simulink model "model"  (R2023b)
settings: Solver=VariableStepAuto  StartTime=0.0  StopTime=10.0  RelTol=1e-3
undefined symbols (not defined in the file): a253, a483c26d3aa4, a58537c8, DiscIntNeverNeededParam, magnitude, Newton, Raphson
libraries: simulink x123, slpidlib x33
(part 1 of 5)
settings Model: Creator=OSCAR4  LastModifiedBy=OSCAR4

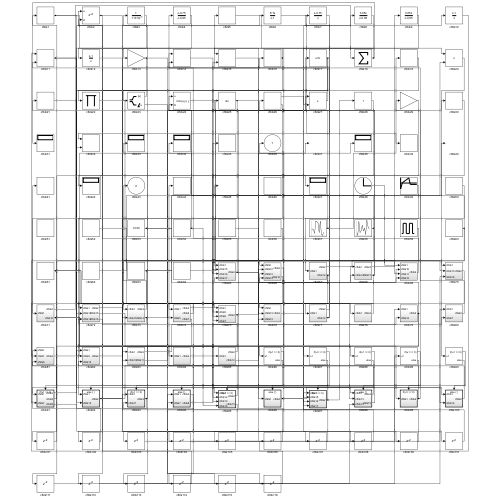
[thumbnail: Simulink's stored preview of the top-level diagram]
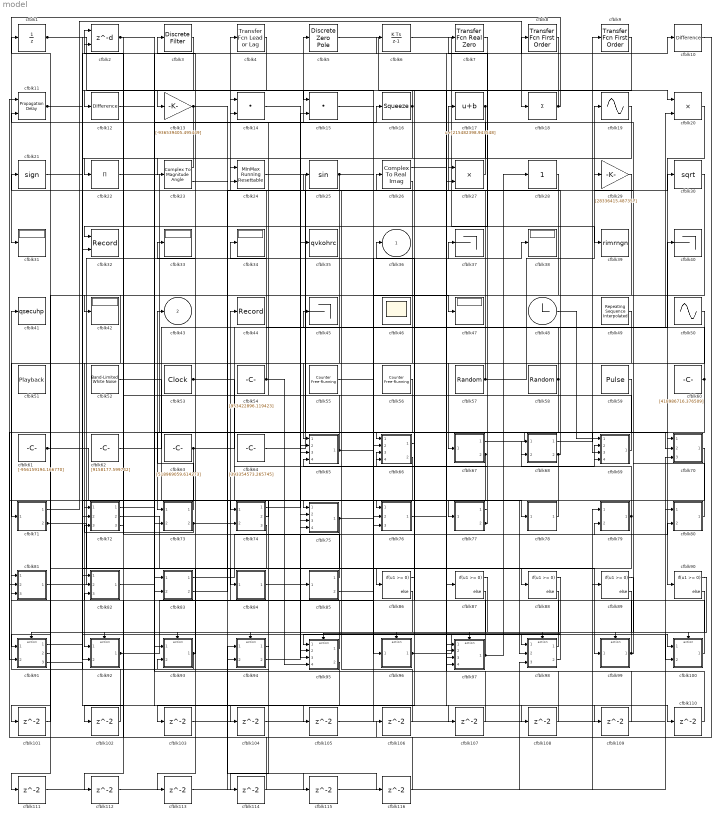
== system model ==
  cfblk1 : UnitDelay  HasFrameUpgradeWarning=on
  cfblk10 : simulink/Discrete/Difference  ICPrevInput=0.0  OutMin=[]  OutMax=[]  OutDataTypeStr=Inherit: Inherit via back propagation  OutDataType=fixdt(1, 16)  OutScaling=2^-10  DoSatur=off
  cfblk100 : Subsystem  TreatAsAtomicUnit=on
  cfblk{101..116} (16 alike) : Delay  SampleTime=1
  cfblk11 : PropagationDelay  SampleTime=1
  cfblk12 : simulink/Discrete/Difference  ICPrevInput=0.0  OutMin=[]  OutMax=[]  OutDataTypeStr=Inherit: Inherit via back propagation  OutDataType=fixdt(1, 16)  OutScaling=2^-10  DoSatur=off
  cfblk13 : Gain  Gain=[-936539405.495449]
  cfblk14 : DotProduct  OutDataTypeStr=Inherit: Inherit via internal rule
  cfblk15 : DotProduct  OutDataTypeStr=Inherit: Inherit via internal rule
  cfblk16 : Squeeze
  cfblk17 : Bias  Bias=[215482398.943548]  SaturateOnIntegerOverflow=off
  cfblk18 : Sum  Inputs=+
  cfblk19 : Sin  TimeSource=Use external signal  SampleTime=0
  cfblk2 : Delay  DelayLengthSource=Input port  SampleTime=1
      settings: InputPortMap=u0,p1
  cfblk20 : Product  Inputs=**
  cfblk21 : Signum
  cfblk22 : Product  Inputs=*
  cfblk23 : ComplexToMagnitudeAngle
  cfblk24 : simulink/Math Operations/MinMax Running Resettable  Function=min  vinit=0.0
  cfblk25 : Trigonometry
  cfblk26 : ComplexToRealImag
  cfblk27 : Product  Inputs=**
  cfblk28 : simulink/Math Operations/Slider Gain  gain=1  low=0  high=2
  cfblk29 : Gain  Gain=[28336415.487357]
  cfblk3 : DiscreteFilter  SampleTime=1
  cfblk30 : Sqrt
  cfblk{31,33..34,38,42,47} (6 alike) : Display
  cfblk32 : Record  FileSettingsInternal="{\"entries\":[{\"content\":{\"excelSettings\":{\"content\":{},\"type\":\"Streamout.ExcelSettings\"}},\"type\":\"Streamout.FileSettingStorage\",\"uuid\":\"\"}],\"packageUris\":[\"http:\\/\\/schema.mathworks.com\\/mf0\\/streamout_blocks\\/R2020a\"],\"version\":\"1.0\"}"  Layout=[1 1]  SignalsInternal="{\"entries\":[{\"content\":{\"signals\":[{\"content\":{\"blockPath\":[],\"dimensions\":[1],\"domain\":\"\",\"lineColor\":\"#a2142f\",\"plots\":[1],\"port\":1,\"signalID\":333,\"signalName\":\"XY Graph:1\"},\"type\":\"RecordBlkView.Signal\",\"uuid\":\"\"},{\"content\":{\"blockPath\":[],\"dimensions\":[1],\"domain\":\"\",\"lineColor\":\"#139fff\",\"plots\":[1],\"port\":2,\"signalID\":336,\"signalName\":\"XY Graph:2\"},\"type\":\"RecordBlkView.Signal\",\"uuid\":\"\"}]},\"type\":\"RecordBlkView.InputSignals\",\"uuid\":\"\"}],\"packageUris\":[\"http:\\/\\/schema.mathworks.com\\/mf0\\/streamout_blocks\\/R2020a\"],\"version\":\"1.0\"}"  VisualizationBindings="{\"xyplotplugin\":{\"info\":[{\"series\":[{\"bindingParametersList\":[{\"parameter\":\"X-Axis\",\"signalID\":333,\"signalName\":\"XY Graph:1\"},{\"parameter\":\"Y-Axis\",\"signalID\":336,\"signalName\":\"XY Graph:2\"}],\"seriesID\":1381}],\"subplotID\":1}]}}"  CompatibilityTag=XY
  cfblk35 : ToWorkspace  VariableName=qvkohrc  SaveFormat=Timeseries  SampleTime=-1
  cfblk37 : Terminator
  cfblk39 : ToWorkspace  VariableName=rimrngn  SaveFormat=Timeseries  SampleTime=-1
  cfblk4 : simulink/Discrete/Transfer Fcn Lead or Lag  PoleZ=0.95  ZeroZ=0.75  ICPrevOutput=0.0  ICPrevInput=0.0  DoSatur=off
  cfblk40 : Terminator
  cfblk41 : ToWorkspace  VariableName=qsecuhp  SaveFormat=Timeseries  SampleTime=-1
  cfblk44 : Record  FileSettingsInternal="{\"entries\":[{\"content\":{\"excelSettings\":{\"content\":{},\"type\":\"Streamout.ExcelSettings\"}},\"type\":\"Streamout.FileSettingStorage\",\"uuid\":\"\"}],\"packageUris\":[\"http:\\/\\/schema.mathworks.com\\/mf0\\/streamout_blocks\\/R2020a\"],\"version\":\"1.0\"}"  SignalsInternal="{\"entries\":[{\"content\":{},\"type\":\"RecordBlkView.InputSignals\",\"uuid\":\"\"}],\"packageUris\":[\"http:\\/\\/schema.mathworks.com\\/mf0\\/streamout_blocks\\/R2020a\"],\"version\":\"1.0\"}"  VisualizationBindings="{\"sparklinesplugin\":{\"info\":[{\"bindingParametersList\":[],\"subplotID\":1}]}}"
  cfblk45 : Terminator
  cfblk46 : Scope
      settings: Floating=on
  cfblk48 : Clock
  cfblk49 : simulink/Sources/Repeating Sequence Interpolated  OutValues=[-862246933.189971, 79795425.555159, 796029637.329822, -177271712.383699, -203597038.742514]  TimeValues=[0 0.1 0.5 0.6 1].'  LookUpMeth=Use Input Above  tsamp=0.01  OutMin=[]  OutMax=[]  OutDataTypeStr=double  OutputDataTypeScalingMode=double  OutDataType=fixdt(0,8)  OutScaling=2^-10
  cfblk5 : DiscreteZeroPole  Poles=[0 0.5]  Gain=1
  cfblk50 : Sin  Amplitude=[622397523.758489]  Bias=[68547005.057914]  SampleTime=0
  cfblk51 : Playback  NumPorts=0  PartName=a58537c8-2575-4d09-a253-a483c26d3aa4
  cfblk52 : simulink/Sources/Band-Limited White Noise  Cov=[7865533069.385715]  Ts=0.1  seed=[9991167842.000000]
  cfblk53 : DigitalClock
  cfblk54 : Constant  Value=[953422896.119423]  SampleTime=1
  cfblk55 : simulink/Sources/Counter Free-Running  NumBits=[8.000000]  tsamp=-1
  cfblk56 : simulink/Sources/Counter Free-Running  NumBits=[25.000000]  tsamp=-1
  cfblk57 : RandomNumber  Mean=[27099.703573]  Variance=[54296.355318]  Seed=[492554018.000000]  SampleTime=0.1
  cfblk58 : UniformRandomNumber  Minimum=[-5476740076.138133]  Maximum=[6087892347.861098]  Seed=[38639628.000000]  SampleTime=0.1
  cfblk59 : DiscretePulseGenerator  PulseType=Time based  Amplitude=[-963513943.362810]  Period=[45867571.560506]  PulseWidth=5  PhaseDelay=[2.000000]
  cfblk6 : DiscreteIntegrator  ICPrevOutput=DiscIntNeverNeededParam  ICPrevScaledInput=DiscIntNeverNeededParam
  cfblk60 : Constant  Value=[418986716.376509]  SampleTime=1
  cfblk61 : Constant  Value=[-956159194.166770]  SampleTime=1
  cfblk62 : Constant  Value=[9158177.599742]  SampleTime=1
  cfblk63 : Constant  Value=[518969059.614273]  SampleTime=1
  cfblk64 : Constant  Value=[393354573.265745]  SampleTime=1
  cfblk65 : Subsystem
  cfblk66 : Subsystem
  cfblk67 : Subsystem
  cfblk68 : Subsystem
  cfblk69 : Subsystem
  cfblk7 : simulink/Discrete/Transfer Fcn Real Zero  ZeroZ=0.75  ICPrevInput=0.0  DoSatur=off
  cfblk70 : Subsystem
  cfblk71 : Subsystem
  cfblk72 : Subsystem
  cfblk73 : Subsystem
  cfblk74 : Subsystem
  cfblk75 : Subsystem
  cfblk76 : Subsystem
  cfblk77 : Subsystem
  cfblk78 : Subsystem
  cfblk79 : Subsystem
  cfblk8 : simulink/Discrete/Transfer Fcn First Order  PoleZ=0.95  ICPrevOutput=0.0  DoSatur=off
  cfblk80 : Subsystem
  cfblk81 : Subsystem
  cfblk82 : Subsystem
  cfblk83 : Subsystem
  cfblk84 : Subsystem
  cfblk85 : Subsystem
  cfblk{86..90} (5 alike) : If  IfExpression=u1 >= 0  SampleTime=1
  cfblk9 : simulink/Discrete/Transfer Fcn First Order  PoleZ=0.95  ICPrevOutput=0.0  DoSatur=off
  cfblk91 : Subsystem  TreatAsAtomicUnit=on
  cfblk92 : Subsystem  TreatAsAtomicUnit=on
  cfblk93 : Subsystem  TreatAsAtomicUnit=on
  cfblk94 : Subsystem  TreatAsAtomicUnit=on
  cfblk95 : Subsystem  TreatAsAtomicUnit=on
  cfblk96 : Subsystem  TreatAsAtomicUnit=on
  cfblk97 : Subsystem  TreatAsAtomicUnit=on
  cfblk98 : Subsystem  TreatAsAtomicUnit=on
  cfblk99 : Subsystem  TreatAsAtomicUnit=on
  cfblk36 : Outport
  cfblk43 : Outport  Port=2
  wires:
  cfblk20/1 -> cfblk90/1
  cfblk81/1(cfblk2) -> cfblk38/1
  cfblk52/1 -> cfblk75/1(cfblk1)
  cfblk27/1 -> cfblk5/1
  cfblk4/1 -> cfblk12/1
  cfblk78/1(cfblk2) -> cfblk76/1(cfblk1)
  cfblk48/1 -> cfblk69/1(cfblk1)
  cfblk7/1 -> cfblk32/1
  cfblk22/1 -> cfblk70/1(cfblk1)
  cfblk57/1 -> cfblk19/1, cfblk14/2
  cfblk99/1(cfblk2) -> cfblk29/1, cfblk81/3(cfblk8)
  cfblk59/1 -> cfblk73/1(cfblk1)
  cfblk14/1 -> cfblk85/1(cfblk1)
  cfblk71/1(cfblk2) -> cfblk18/1
  cfblk82/1(cfblk2) -> cfblk16/1
  cfblk95/1(cfblk2) -> cfblk44/1
  cfblk16/1 -> cfblk13/1, cfblk65/2(cfblk15)
  cfblk55/1 -> cfblk96/1(cfblk1)
  cfblk18/1 -> cfblk31/1, cfblk15/1
  cfblk6/1 -> cfblk39/1
  cfblk70/1(cfblk2) -> cfblk83/2(cfblk10)
  cfblk19/1 -> cfblk42/1
  cfblk58/1 -> cfblk4/1, cfblk91/1(cfblk1)
  cfblk30/1 -> cfblk92/1(cfblk1)
  cfblk24/1 -> cfblk66/1(cfblk1)
  cfblk93/1(cfblk2) -> cfblk41/1, cfblk3/1
  cfblk92/1(cfblk2) -> cfblk66/2(cfblk12), cfblk6/1, cfblk108/1
  cfblk75/1(cfblk2) -> cfblk69/4(cfblk12), cfblk114/1
  cfblk13/1 -> cfblk23/1, cfblk116/1
  cfblk97/1(cfblk2) -> cfblk25/1, cfblk28/1
  cfblk96/1(cfblk2) -> cfblk98/1(cfblk1), cfblk8/1
  cfblk3/1 -> cfblk32/2
  cfblk9/1 -> cfblk86/1
  cfblk91/1(cfblk2) -> cfblk10/1
  cfblk60/1 -> cfblk34/1, cfblk95/3(cfblk13), cfblk65/3(cfblk16)
  cfblk79/1(cfblk2) -> cfblk82/2(cfblk9), cfblk68/1(cfblk1), cfblk101/1
  cfblk1/1 -> cfblk76/2(cfblk13), cfblk75/3(cfblk6)
  cfblk15/1 -> cfblk47/1
  cfblk64/1 -> cfblk17/1
  cfblk68/1(cfblk2) -> cfblk9/1
  cfblk74/1(cfblk2) -> cfblk35/1
  cfblk67/1(cfblk2) -> cfblk70/2(cfblk15)
  cfblk49/1 -> cfblk71/1(cfblk1)
  cfblk12/1 -> cfblk100/1(cfblk1)
  cfblk80/1(cfblk2) -> cfblk11/2
  cfblk98/1(cfblk2) -> cfblk33/1
  cfblk68/2(cfblk15) -> cfblk26/1, cfblk74/2(cfblk5), cfblk21/1
  cfblk85/1(cfblk2) -> cfblk2/1
  cfblk23/1 -> cfblk22/1
  cfblk5/1 -> cfblk20/1
  cfblk100/1(cfblk2) -> cfblk36/1
  cfblk63/1 -> cfblk40/1, cfblk66/4(cfblk14), cfblk91/2(cfblk7)
  cfblk69/1(cfblk2) -> cfblk24/1
  cfblk71/2(cfblk10) -> cfblk88/1, cfblk95/2(cfblk12)
  cfblk98/2(cfblk15) -> cfblk95/1(cfblk1)
  cfblk17/1 -> cfblk92/2(cfblk13), cfblk72/2(cfblk13)
  cfblk85/2(cfblk12) -> cfblk69/2(cfblk10)
  cfblk74/2(cfblk6) -> cfblk72/1(cfblk1)
  cfblk53/1 -> cfblk98/2(cfblk13), cfblk15/2
  cfblk62/1 -> cfblk20/2
  cfblk28/1 -> cfblk75/2(cfblk5)
  cfblk72/2(cfblk15) -> cfblk99/1(cfblk1)
  cfblk25/1 -> cfblk77/1(cfblk1), cfblk65/1(cfblk1)
  cfblk11/1 -> cfblk84/1(cfblk1), cfblk97/4(cfblk17)
  cfblk61/1 -> cfblk78/1(cfblk1), cfblk75/4(cfblk7)
  cfblk91/2(cfblk8) -> cfblk81/1(cfblk1)
  cfblk67/2(cfblk12) -> cfblk66/3(cfblk13), cfblk45/1, cfblk97/3(cfblk16)
  cfblk77/1(cfblk2) -> cfblk7/1
  cfblk83/1(cfblk2) -> cfblk80/2(cfblk7)
  cfblk50/1 -> cfblk67/1(cfblk1)
  cfblk2/1 -> cfblk69/3(cfblk11), cfblk102/1
  cfblk83/2(cfblk11) -> cfblk27/1
  cfblk8/1 -> cfblk27/2
  cfblk73/1(cfblk2) -> cfblk43/1
  cfblk21/1 -> cfblk74/1(cfblk1)
  cfblk65/1(cfblk2) -> cfblk2/2, cfblk37/1, cfblk68/2(cfblk14)
  cfblk76/1(cfblk2) -> cfblk87/1
  cfblk56/1 -> cfblk81/2(cfblk7)
  cfblk26/2 -> cfblk73/2(cfblk11)
  cfblk94/1(cfblk2) -> cfblk93/2(cfblk11)
  cfblk77/2(cfblk12) -> cfblk14/1, cfblk65/4(cfblk17)
  cfblk54/1 -> cfblk24/2, cfblk95/4(cfblk14)
  cfblk73/2(cfblk12) -> cfblk30/1, cfblk72/3(cfblk14)
  cfblk84/1(cfblk2) -> cfblk100/2(cfblk14)
  cfblk94/2(cfblk8) -> cfblk79/2(cfblk14)
  cfblk86/1 -> cfblk91/Action
  cfblk86/2 -> cfblk92/Action
  cfblk87/1 -> cfblk93/Action
  cfblk87/2 -> cfblk94/Action
  cfblk88/1 -> cfblk95/Action
  cfblk88/2 -> cfblk96/Action
  cfblk89/1 -> cfblk97/Action
  cfblk89/2 -> cfblk98/Action
  cfblk90/1 -> cfblk99/Action
  cfblk90/2 -> cfblk100/Action
  cfblk101/1 -> cfblk1/1
  cfblk102/1 -> cfblk82/1(cfblk1)
  cfblk66/1(cfblk2) -> cfblk103/1
  cfblk103/1 -> cfblk80/1(cfblk1)
  cfblk66/2(cfblk15) -> cfblk104/1
  cfblk104/1 -> cfblk89/1
  cfblk95/2(cfblk15) -> cfblk105/1
  cfblk105/1 -> cfblk76/3(cfblk14)
  cfblk10/1 -> cfblk106/1
  cfblk106/1 -> cfblk83/1(cfblk1)
  cfblk91/3(cfblk9) -> cfblk107/1
  cfblk107/1 -> cfblk93/1(cfblk1)
  cfblk108/1 -> cfblk97/2(cfblk15)
  cfblk26/1 -> cfblk109/1
  cfblk109/1 -> cfblk97/1(cfblk1)
  cfblk72/1(cfblk2) -> cfblk110/1
  cfblk110/1 -> cfblk94/1(cfblk1)
  cfblk29/1 -> cfblk111/1
  cfblk111/1 -> cfblk98/3(cfblk14)
  cfblk72/3(cfblk16) -> cfblk112/1
  cfblk112/1 -> cfblk70/3(cfblk16)
  cfblk74/3(cfblk7) -> cfblk113/1
  cfblk113/1 -> cfblk94/2(cfblk7)
  cfblk114/1 -> cfblk11/1
  cfblk23/2 -> cfblk115/1
  cfblk115/1 -> cfblk79/1(cfblk1)
  cfblk116/1 -> cfblk82/3(cfblk10)

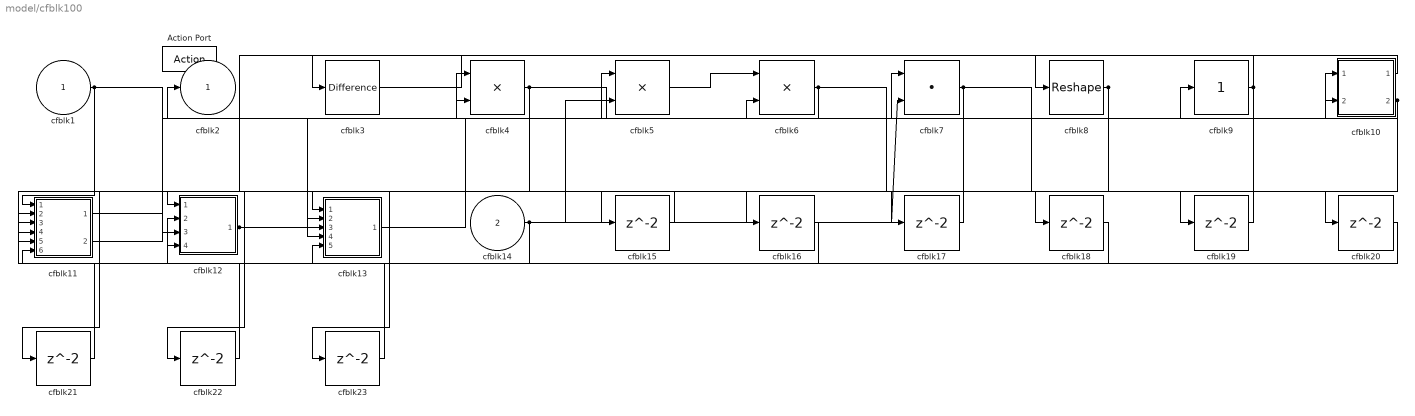
== system model/cfblk100 ==
  cfblk1 : Inport
  cfblk14 : Inport  Port=2
  Action Port : ActionPort  ActionPortLabel=else
  cfblk10 : Subsystem
  cfblk11 : Subsystem
  cfblk12 : Subsystem
  cfblk13 : Subsystem
  cfblk{15..23} (9 alike) : Delay
  cfblk3 : simulink/Discrete/Difference  ICPrevInput=0.0  OutMin=[]  OutMax=[]  OutDataTypeStr=Inherit: Inherit via back propagation  OutDataType=fixdt(1, 16)  OutScaling=2^-10  DoSatur=off
  cfblk4 : Product  Inputs=**
  cfblk5 : Product
  cfblk6 : Product
  cfblk7 : DotProduct  OutDataTypeStr=Inherit: Inherit via internal rule
  cfblk8 : Reshape
  cfblk9 : simulink/Math Operations/Slider Gain  gain=1  low=0  high=2
  cfblk2 : Outport
  wires:
  cfblk13/1(cfblk2) -> cfblk10/1(cfblk1)
  cfblk9/1 -> cfblk12/1(cfblk1), cfblk12/3(cfblk7)
  cfblk14/1 -> cfblk12/2(cfblk6), cfblk5/2, cfblk7/2
  cfblk11/1(cfblk2) -> cfblk9/1
  cfblk7/1 -> cfblk13/1(cfblk1), cfblk20/1
  cfblk10/1(cfblk2) -> cfblk3/1
  cfblk1/1 -> cfblk11/1(cfblk1), cfblk4/1
  cfblk6/1 -> cfblk2/1, cfblk18/1, cfblk19/1
  cfblk11/2(cfblk15) -> cfblk10/2(cfblk16)
  cfblk10/2(cfblk17) -> cfblk5/1, cfblk17/1
  cfblk12/1(cfblk2) -> cfblk7/1, cfblk4/2
  cfblk5/1 -> cfblk6/1
  cfblk8/1 -> cfblk15/1, cfblk16/1
  cfblk3/1 -> cfblk8/1
  cfblk4/1 -> cfblk6/2, cfblk13/4(cfblk16), cfblk21/1, cfblk22/1, cfblk23/1
  cfblk15/1 -> cfblk13/3(cfblk15)
  cfblk16/1 -> cfblk12/4(cfblk8)
  cfblk17/1 -> cfblk13/2(cfblk14)
  cfblk18/1 -> cfblk13/5(cfblk17)
  cfblk19/1 -> cfblk11/3(cfblk11)
  cfblk20/1 -> cfblk11/5(cfblk13)
  cfblk21/1 -> cfblk11/2(cfblk10)
  cfblk22/1 -> cfblk11/4(cfblk12)
  cfblk23/1 -> cfblk11/6(cfblk14)

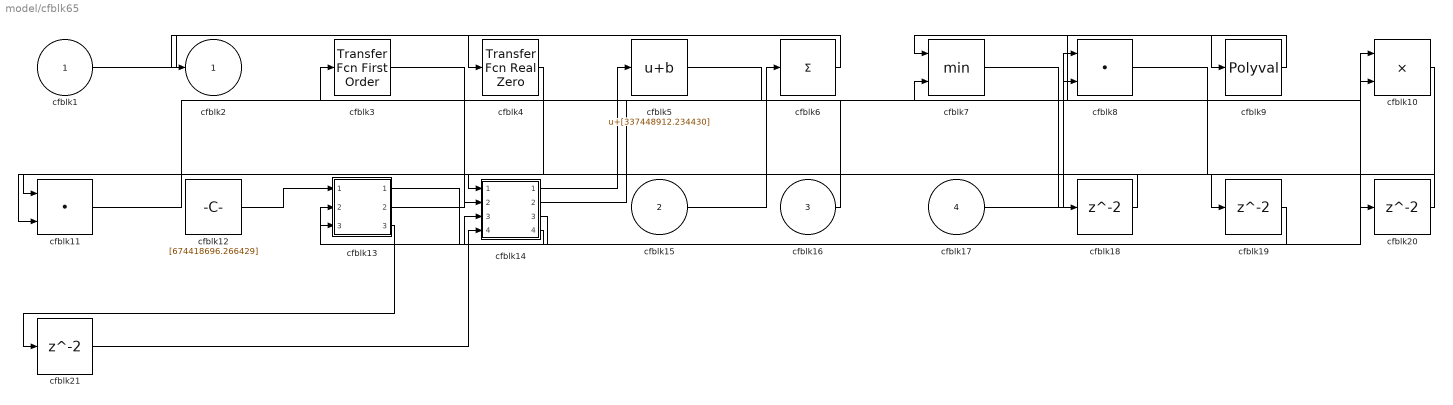
== system model/cfblk65 ==
  cfblk1 : Inport
  cfblk15 : Inport  Port=2
  cfblk16 : Inport  Port=3
  cfblk17 : Inport  Port=4
  cfblk10 : Product
  cfblk11 : DotProduct  OutDataTypeStr=Inherit: Inherit via internal rule
  cfblk12 : Constant  Value=[674418696.266429]  SampleTime=1
  cfblk13 : Subsystem
  cfblk14 : Subsystem
  cfblk{18..21} (4 alike) : Delay  SampleTime=1
  cfblk3 : simulink/Discrete/Transfer Fcn First Order  PoleZ=0.95  ICPrevOutput=0.0  DoSatur=off
  cfblk4 : simulink/Discrete/Transfer Fcn Real Zero  ZeroZ=0.75  ICPrevInput=0.0  DoSatur=off
  cfblk5 : Bias  Bias=[337448912.234430]  SaturateOnIntegerOverflow=off
  cfblk6 : Sum  Inputs=+
  cfblk7 : MinMax  Inputs=2
  cfblk8 : DotProduct  OutDataTypeStr=Inherit: Inherit via internal rule
  cfblk9 : Polyval  Coefs=[ +2.081618890e-019, -1.441693666e-014, +4.719686976e-010, -8.536869453e-006, +1.621573104e-001, -8.087801117e+001 ]
  cfblk2 : Outport
  wires:
  cfblk1/1 -> cfblk4/1
  cfblk11/1 -> cfblk9/1
  cfblk14/1(cfblk2) -> cfblk5/1
  cfblk13/1(cfblk2) -> cfblk10/1
  cfblk6/1 -> cfblk2/1
  cfblk16/1 -> cfblk3/1
  cfblk4/1 -> cfblk11/2
  cfblk15/1 -> cfblk6/1
  cfblk9/1 -> cfblk7/1
  cfblk3/1 -> cfblk14/2(cfblk10)
  cfblk5/1 -> cfblk10/2
  cfblk12/1 -> cfblk13/1(cfblk1)
  cfblk13/2(cfblk14) -> cfblk7/2
  cfblk14/2(cfblk13) -> cfblk8/1
  cfblk17/1 -> cfblk8/2
  cfblk14/3(cfblk14) -> cfblk13/2(cfblk12)
  cfblk14/4(cfblk15) -> cfblk13/3(cfblk13)
  cfblk7/1 -> cfblk18/1
  cfblk18/1 -> cfblk11/1
  cfblk10/1 -> cfblk19/1
  cfblk19/1 -> cfblk14/3(cfblk11)
  cfblk8/1 -> cfblk20/1
  cfblk20/1 -> cfblk14/1(cfblk1)
  cfblk13/3(cfblk15) -> cfblk21/1
  cfblk21/1 -> cfblk14/4(cfblk12)

== system model/cfblk66 ==
  cfblk1 : Inport
  cfblk12 : Inport  Port=2
  cfblk13 : Inport  Port=3
  cfblk14 : Inport  Port=4
  cfblk10 : Subsystem
  cfblk11 : Subsystem
  cfblk16 : Delay  SampleTime=1
  cfblk3 : PropagationDelay  SampleTime=1
  cfblk4 : ComplexToRealImag
  cfblk5 : Product  Inputs=*
  cfblk6 : Trigonometry
  cfblk7 : Constant  Value=[628183486.568107]  SampleTime=1
  cfblk8 : Constant  Value=[532735345.573752]  SampleTime=1
  cfblk9 : Subsystem
  cfblk2 : Outport
  cfblk15 : Outport  Port=2
  wires:
  cfblk12/1 -> cfblk11/1(cfblk1)
  cfblk8/1 -> cfblk2/1
  cfblk10/1(cfblk2) -> cfblk5/1
  cfblk3/1 -> cfblk10/1(cfblk1)
  cfblk6/1 -> cfblk4/1
  cfblk14/1 -> cfblk15/1
  cfblk7/1 -> cfblk3/1
  cfblk9/1(cfblk2) -> cfblk6/1
  cfblk5/1 -> cfblk9/1(cfblk1)
  cfblk11/1(cfblk2) -> cfblk3/2
  cfblk1/1 -> cfblk9/2(cfblk12)
  cfblk11/2(cfblk14) -> cfblk9/3(cfblk13)
  cfblk13/1 -> cfblk9/5(cfblk15)
  cfblk4/1 -> cfblk16/1
  cfblk16/1 -> cfblk9/4(cfblk14)

== system model/cfblk67 ==
  cfblk1 : Inport
  cfblk10 : Subsystem
  cfblk11 : Subsystem
  cfblk13 : Delay  SampleTime=1
  cfblk14 : Delay  SampleTime=1
  cfblk15 : Delay  SampleTime=1
  cfblk3 : simulink/Discrete/Tapped Delay  vinit=0.0  samptime=-1  NumDelays=1  DelayOrder=Oldest  includeCurrent=off
  cfblk4 : simulink/Discrete/Difference  ICPrevInput=0.0  OutMin=[]  OutMax=[]  OutDataTypeStr=Inherit: Inherit via back propagation  OutDataType=fixdt(1, 16)  OutScaling=2^-10  DoSatur=off
  cfblk5 : simulink/Discrete/Transfer Fcn Lead or Lag  PoleZ=0.95  ZeroZ=0.75  ICPrevOutput=0.0  ICPrevInput=0.0  DoSatur=off
  cfblk6 : Signum
  cfblk7 : Sum
  cfblk8 : simulink/Math Operations/MinMax Running Resettable  Function=min  vinit=0.0
  cfblk9 : Constant  Value=[-707875031.415103]  SampleTime=1
  cfblk2 : Outport
  cfblk12 : Outport  Port=2
  wires:
  cfblk7/1 -> cfblk6/1, cfblk14/1
  cfblk3/1 -> cfblk7/1
  cfblk10/1(cfblk2) -> cfblk2/1
  cfblk8/1 -> cfblk3/1, cfblk15/1
  cfblk11/1(cfblk2) -> cfblk8/1
  cfblk9/1 -> cfblk7/2
  cfblk10/2(cfblk13) -> cfblk8/2
  cfblk1/1 -> cfblk5/1, cfblk10/3(cfblk10)
  cfblk10/3(cfblk14) -> cfblk12/1
  cfblk4/1 -> cfblk10/2(cfblk9), cfblk11/2(cfblk7)
  cfblk5/1 -> cfblk4/1, cfblk11/1(cfblk1)
  cfblk6/1 -> cfblk13/1
  cfblk13/1 -> cfblk10/1(cfblk1)
  cfblk14/1 -> cfblk10/5(cfblk12)
  cfblk15/1 -> cfblk10/4(cfblk11)

== system model/cfblk68 ==
  cfblk1 : Inport
  cfblk14 : Inport  Port=2
  cfblk10 : Constant  Value=[-460195986.517128]  SampleTime=1
  cfblk11 : Constant  Value=[291746783.865006]  SampleTime=1
  cfblk12 : Subsystem
  cfblk13 : Subsystem
  cfblk16 : Delay  SampleTime=1
  cfblk17 : Delay  SampleTime=1
  cfblk3 : Delay  ShowEnablePort=on  SampleTime=1
      settings: InputPortMap=u0,e6
  cfblk4 : slpidlib/PID Controller  Controller=PID  Form=Parallel  TimeDomain=Discrete-time  UseExternalTs=off  SampleTime=1  IntegratorMethod=Forward Euler  FilterMethod=Forward Euler  ControllerParametersSource=internal  P=1  I=1  UseKiTs=off  D=0  N=100  UseFilter=on  TunerSelectOption=Transfer Function Based (PID Tuner App)  InitialConditionSource=internal  InitialConditionForIntegrator=0  InitialConditionForFilter=0  DifferentiatorICPrevScaledInput=0  ExternalReset=none  TrackingMode=off  Kt=1  LimitOutput=off  SatLimitsSource=internal  UpperSaturationLimit=inf  LowerSaturationLimit=-inf  LinearizeAsGain=off  AntiWindupMode=none  Kb=1  LimitIntegrator=off  UpperIntegratorSaturationLimit=inf  LowerIntegratorSaturationLimit=-inf  POutMin=[]  POutMax=[]  IOutMin=[]  IOutMax=[]  DOutMin=[]  DOutMax=[]  NOutMin=[]  NOutMax=[]  SumOutMin=[]  SumOutMax=[]  SaturationOutMin=[]  SaturationOutMax=[]  PParamMin=[]  PParamMax=[]  IParamMin=[]  IParamMax=[]  DParamMin=[]  DParamMax=[]  NParamMin=[]  NParamMax=[]  KbParamMin=[]  KbParamMax=[]  KtParamMin=[]  KtParamMax=[]  KbOutMin=[]  KbOutMax=[]  KtOutMin=[]  KtOutMax=[]  IntegratorOutMin=[]  IntegratorOutMax=[]  FilterOutMin=[]  FilterOutMax=[]  SumI1OutMin=[]  SumI1OutMax=[]  SumI2OutMin=[]  SumI2OutMax=[]  SumI3OutMin=[]  SumI3OutMax=[]  SumI4OutMin=[]  SumI4OutMax=[]  SumDOutMin=[]  SumDOutMax=[]  DifferentiatorOutMin=[]  DifferentiatorOutMax=[]  FilterDiffOutCoefMin=[]  FilterDiffOutCoefMax=[]  ReciprocalOutMin=[]  ReciprocalOutMax=[]  SumDenOutMin=[]  SumDenOutMax=[]  SumNumOutMin=[]  SumNumOutMax=[]  DivideOutMin=[]  DivideOutMax=[]  UdiffTsProdOutMin=[]  UdiffTsProdOutMax=[]  NTsProdOutMin=[]  NTsProdOutMax=[]  UintegralTsProdOutMin=[]  UintegralTsProdOutMax=[]  UngainTsProdOutMin=[]  UngainTsProdOutMax=[]  ClampingZeroOutDataTypeStr=Inherit: Inherit via back propagation  ClampingZeroOutMin=[]  ClampingZeroOutMax=[]  FilterDenConstantOutDataTypeStr=Inherit: Inherit via back propagation  FilterDenConstantOutMin=[]  FilterDenConstantOutMax=[]  PCopyOutDataTypeStr=Inherit: Inherit via back propagation  PCopyOutMin=[]  PCopyOutMax=[]  NCopyOutDataTypeStr=Inherit: Inherit via back propagation  NCopyOutMin=[]  NCopyOutMax=[]  IntegratorContinuousStateAttributes=''  IntegratorStateMustResolveToSignalObject=off  IntegratorRTWStateStorageClass=Auto  FilterContinuousStateAttributes=''  FilterStateMustResolveToSignalObject=off  FilterRTWStateStorageClass=Auto  ParallelPVariant=InternalParameters  IdealPVariant=Disabled  IVariant=InternalParameters  DVariant=InternalParameters  IntegratorVariant=Discrete  SatVariant=Disabled  AWVariant=Passthrough  PCopyVariant=Disabled  TRVariant=Disabled  FdbkBlocksVariant=Forward  IdealPFdbkVariant=Disabled  SatFdbkVariant=Disabled  DerivativeFilterVariant=ForwardEulerFilter  NVariant=InternalParameters  NCopyVariant=Disabled  FilterICVariant=InternalICsFilter  IntegratorICVariant=InternalICs  ExternalResetVariant=Disabled  TRSumVariant=Passthrough  SumFdbkVariant=Disabled  SumVariant=Sum_PID  TsampFilterVariant=InternalTs  TsampNgainVariant=Passthrough  TsampIntegralVariant=Disabled_SignalSpec  ExternalSaturationOutDataTypeStr=Inherit: Same as second input
      settings: LibrarySourceBlock=simulink/Discrete/Discrete PID Controller
  cfblk5 : PropagationDelay  SampleTime=1
  cfblk6 : DotProduct  OutDataTypeStr=Inherit: Inherit via internal rule
  cfblk7 : DotProduct  OutDataTypeStr=Inherit: Inherit via internal rule
  cfblk8 : Sqrt  Operator=rSqrt  AlgorithmType=Newton-Raphson
  cfblk9 : Sqrt  Operator=rSqrt  AlgorithmType=Newton-Raphson
  cfblk2 : Outport
  cfblk15 : Outport  Port=2
  wires:
  cfblk3/1 -> cfblk8/1
  cfblk13/1(cfblk2) -> cfblk12/1(cfblk1)
  cfblk8/1 -> cfblk15/1
  cfblk10/1 -> cfblk12/2(cfblk10)
  cfblk13/2(cfblk9) -> cfblk5/1
  cfblk14/1 -> cfblk9/1
  cfblk9/1 -> cfblk2/1, cfblk6/2
  cfblk11/1 -> cfblk4/1, cfblk13/3(cfblk8)
  cfblk1/1 -> cfblk7/1
  cfblk6/1 -> cfblk3/1
  cfblk4/1 -> cfblk7/2
  cfblk7/1 -> cfblk13/1(cfblk1), cfblk13/2(cfblk7), cfblk3/2
  cfblk5/1 -> cfblk16/1, cfblk17/1
  cfblk12/1(cfblk2) -> cfblk5/2
  cfblk12/2(cfblk13) -> cfblk6/1
  cfblk16/1 -> cfblk12/3(cfblk11)
  cfblk17/1 -> cfblk12/4(cfblk12)

== system model/cfblk69 ==
  cfblk1 : Inport
  cfblk10 : Inport  Port=2
  cfblk11 : Inport  Port=3
  cfblk12 : Inport  Port=4
  cfblk{13..16} (4 alike) : Delay  SampleTime=1
  cfblk3 : slpidlib/PID Controller  Controller=PID  Form=Parallel  TimeDomain=Discrete-time  UseExternalTs=off  SampleTime=1  IntegratorMethod=Forward Euler  FilterMethod=Forward Euler  ControllerParametersSource=internal  P=1  I=1  UseKiTs=off  D=0  N=100  UseFilter=on  TunerSelectOption=Transfer Function Based (PID Tuner App)  InitialConditionSource=internal  InitialConditionForIntegrator=0  InitialConditionForFilter=0  DifferentiatorICPrevScaledInput=0  ExternalReset=none  TrackingMode=off  Kt=1  LimitOutput=off  SatLimitsSource=internal  UpperSaturationLimit=inf  LowerSaturationLimit=-inf  LinearizeAsGain=off  AntiWindupMode=none  Kb=1  LimitIntegrator=off  UpperIntegratorSaturationLimit=inf  LowerIntegratorSaturationLimit=-inf  POutMin=[]  POutMax=[]  IOutMin=[]  IOutMax=[]  DOutMin=[]  DOutMax=[]  NOutMin=[]  NOutMax=[]  SumOutMin=[]  SumOutMax=[]  SaturationOutMin=[]  SaturationOutMax=[]  PParamMin=[]  PParamMax=[]  IParamMin=[]  IParamMax=[]  DParamMin=[]  DParamMax=[]  NParamMin=[]  NParamMax=[]  KbParamMin=[]  KbParamMax=[]  KtParamMin=[]  KtParamMax=[]  KbOutMin=[]  KbOutMax=[]  KtOutMin=[]  KtOutMax=[]  IntegratorOutMin=[]  IntegratorOutMax=[]  FilterOutMin=[]  FilterOutMax=[]  SumI1OutMin=[]  SumI1OutMax=[]  SumI2OutMin=[]  SumI2OutMax=[]  SumI3OutMin=[]  SumI3OutMax=[]  SumI4OutMin=[]  SumI4OutMax=[]  SumDOutMin=[]  SumDOutMax=[]  DifferentiatorOutMin=[]  DifferentiatorOutMax=[]  FilterDiffOutCoefMin=[]  FilterDiffOutCoefMax=[]  ReciprocalOutMin=[]  ReciprocalOutMax=[]  SumDenOutMin=[]  SumDenOutMax=[]  SumNumOutMin=[]  SumNumOutMax=[]  DivideOutMin=[]  DivideOutMax=[]  UdiffTsProdOutMin=[]  UdiffTsProdOutMax=[]  NTsProdOutMin=[]  NTsProdOutMax=[]  UintegralTsProdOutMin=[]  UintegralTsProdOutMax=[]  UngainTsProdOutMin=[]  UngainTsProdOutMax=[]  ClampingZeroOutDataTypeStr=Inherit: Inherit via back propagation  ClampingZeroOutMin=[]  ClampingZeroOutMax=[]  FilterDenConstantOutDataTypeStr=Inherit: Inherit via back propagation  FilterDenConstantOutMin=[]  FilterDenConstantOutMax=[]  PCopyOutDataTypeStr=Inherit: Inherit via back propagation  PCopyOutMin=[]  PCopyOutMax=[]  NCopyOutDataTypeStr=Inherit: Inherit via back propagation  NCopyOutMin=[]  NCopyOutMax=[]  IntegratorContinuousStateAttributes=''  IntegratorStateMustResolveToSignalObject=off  IntegratorRTWStateStorageClass=Auto  FilterContinuousStateAttributes=''  FilterStateMustResolveToSignalObject=off  FilterRTWStateStorageClass=Auto  ParallelPVariant=InternalParameters  IdealPVariant=Disabled  IVariant=InternalParameters  DVariant=InternalParameters  IntegratorVariant=Discrete  SatVariant=Disabled  AWVariant=Passthrough  PCopyVariant=Disabled  TRVariant=Disabled  FdbkBlocksVariant=Forward  IdealPFdbkVariant=Disabled  SatFdbkVariant=Disabled  DerivativeFilterVariant=ForwardEulerFilter  NVariant=InternalParameters  NCopyVariant=Disabled  FilterICVariant=InternalICsFilter  IntegratorICVariant=InternalICs  ExternalResetVariant=Disabled  TRSumVariant=Passthrough  SumFdbkVariant=Disabled  SumVariant=Sum_PID  TsampFilterVariant=InternalTs  TsampNgainVariant=Passthrough  TsampIntegralVariant=Disabled_SignalSpec  ExternalSaturationOutDataTypeStr=Inherit: Same as second input
      settings: LibrarySourceBlock=simulink/Discrete/Discrete PID Controller
  cfblk4 : Math  Operator=log
  cfblk5 : Trigonometry
  cfblk6 : UnaryMinus
  cfblk7 : Subsystem
  cfblk8 : Subsystem
  cfblk9 : Subsystem
  cfblk2 : Outport
  wires:
  cfblk3/1 -> cfblk6/1
  cfblk7/1(cfblk2) -> cfblk2/1
  cfblk11/1 -> cfblk7/1(cfblk1)
  cfblk12/1 -> cfblk7/2(cfblk9)
  cfblk8/1(cfblk2) -> cfblk3/1
  cfblk10/1 -> cfblk8/1(cfblk1)
  cfblk5/1 -> cfblk4/1
  cfblk8/2(cfblk12) -> cfblk9/1(cfblk1)
  cfblk9/1(cfblk2) -> cfblk5/1
  cfblk1/1 -> cfblk8/5(cfblk11)
  cfblk4/1 -> cfblk7/3(cfblk10)
  cfblk6/1 -> cfblk13/1
  cfblk13/1 -> cfblk8/2(cfblk8)
  cfblk7/2(cfblk11) -> cfblk14/1
  cfblk14/1 -> cfblk9/2(cfblk12)
  cfblk9/2(cfblk13) -> cfblk15/1
  cfblk15/1 -> cfblk8/3(cfblk9)
  cfblk9/3(cfblk14) -> cfblk16/1
  cfblk16/1 -> cfblk8/4(cfblk10)

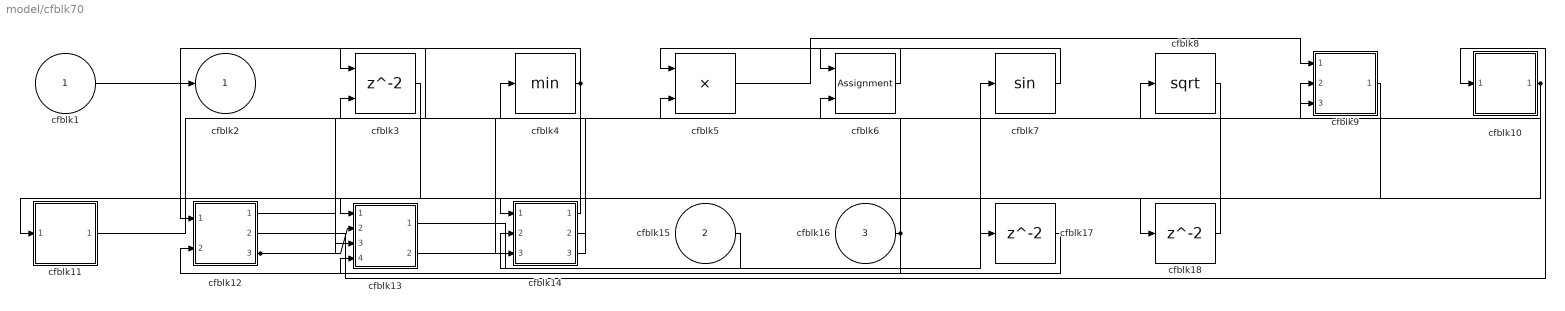
== system model/cfblk70 ==
  cfblk1 : Inport
  cfblk15 : Inport  Port=2
  cfblk16 : Inport  Port=3
  cfblk10 : Subsystem
  cfblk11 : Subsystem
  cfblk12 : Subsystem
  cfblk13 : Subsystem
  cfblk14 : Subsystem
  cfblk17 : Delay  SampleTime=1
  cfblk18 : Delay  SampleTime=1
  cfblk3 : Delay  ShowEnablePort=on  SampleTime=1
      settings: InputPortMap=u0,e6
  cfblk4 : MinMax
  cfblk5 : Product
  cfblk6 : Assignment  DiagnosticForDimensions=Warning  IndexOptions=Index vector (dialog)  Indices=1  OutputSizes=1
  cfblk7 : Trigonometry
  cfblk8 : Sqrt
  cfblk9 : Subsystem
  cfblk2 : Outport
  wires:
  cfblk3/1 -> cfblk11/1(cfblk1)
  cfblk14/1(cfblk2) -> cfblk3/1
  cfblk7/1 -> cfblk6/1
  cfblk13/1(cfblk2) -> cfblk7/1
  cfblk11/1(cfblk2) -> cfblk6/2
  cfblk16/1 -> cfblk3/2, cfblk13/4(cfblk12)
  cfblk1/1 -> cfblk12/1(cfblk1)
  cfblk4/1 -> cfblk2/1, cfblk13/3(cfblk11)
  cfblk13/2(cfblk13) -> cfblk8/1
  cfblk15/1 -> cfblk14/2(cfblk12)
  cfblk10/1(cfblk2) -> cfblk14/3(cfblk13), cfblk5/2
  cfblk5/1 -> cfblk9/1(cfblk1)
  cfblk14/2(cfblk14) -> cfblk4/1
  cfblk6/1 -> cfblk5/1
  cfblk14/3(cfblk15) -> cfblk13/1(cfblk1)
  cfblk12/1(cfblk2) -> cfblk9/2(cfblk10)
  cfblk12/2(cfblk10) -> cfblk10/1(cfblk1)
  cfblk12/3(cfblk11) -> cfblk13/2(cfblk10), cfblk9/3(cfblk11)
  cfblk9/1(cfblk2) -> cfblk17/1
  cfblk17/1 -> cfblk12/2(cfblk9)
  cfblk8/1 -> cfblk18/1
  cfblk18/1 -> cfblk14/1(cfblk1)

== system model/cfblk71 ==
  cfblk1 : Inport
  cfblk{11..14} (4 alike) : Delay  SampleTime=1
  cfblk3 : DiscreteIntegrator  ICPrevOutput=DiscIntNeverNeededParam  ICPrevScaledInput=DiscIntNeverNeededParam
  cfblk4 : ComplexToRealImag
  cfblk5 : Sin  TimeSource=Use external signal  SampleTime=0
  cfblk6 : DotProduct  OutDataTypeStr=Inherit: Inherit via internal rule
  cfblk7 : UnaryMinus
  cfblk8 : Subsystem
  cfblk9 : Subsystem
  cfblk2 : Outport
  cfblk10 : Outport  Port=2
  wires:
  cfblk5/1 -> cfblk12/1, cfblk13/1
  cfblk3/1 -> cfblk4/1
  cfblk8/1(cfblk2) -> cfblk10/1
  cfblk6/1 -> cfblk5/1, cfblk3/1
  cfblk7/1 -> cfblk9/1(cfblk1)
  cfblk1/1 -> cfblk7/1
  cfblk8/3(cfblk14) -> cfblk6/2
  cfblk4/2 -> cfblk2/1
  cfblk9/1(cfblk2) -> cfblk8/1(cfblk1)
  cfblk9/2(cfblk15) -> cfblk8/2(cfblk11)
  cfblk8/2(cfblk13) -> cfblk11/1
  cfblk11/1 -> cfblk9/2(cfblk13)
  cfblk12/1 -> cfblk6/1
  cfblk13/1 -> cfblk8/3(cfblk12)
  cfblk4/1 -> cfblk14/1
  cfblk14/1 -> cfblk9/3(cfblk14)

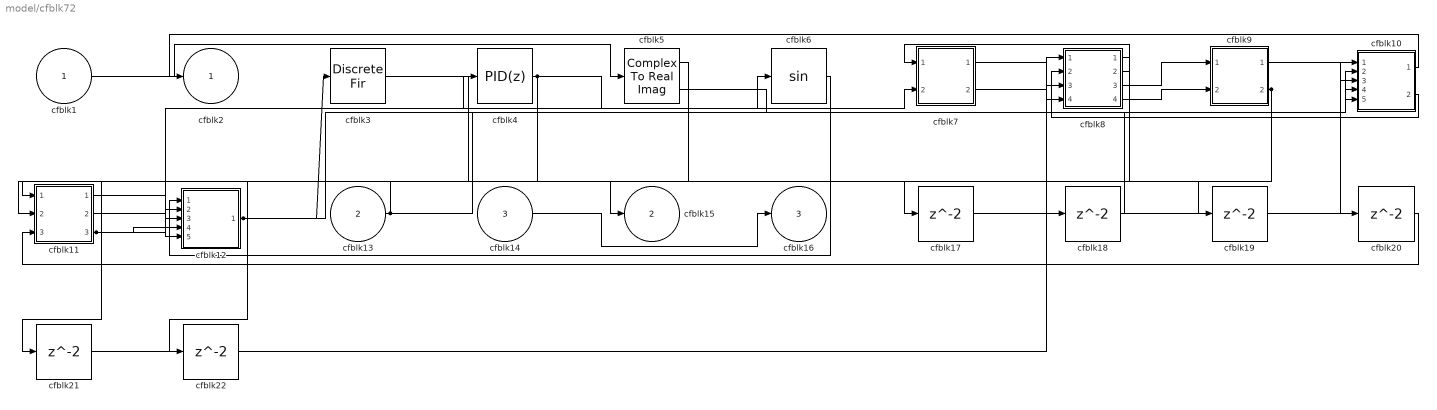
== system model/cfblk72 ==
  cfblk1 : Inport
  cfblk13 : Inport  Port=2
  cfblk14 : Inport  Port=3
  cfblk10 : Subsystem
  cfblk11 : Subsystem
  cfblk12 : Subsystem
  cfblk{17..22} (6 alike) : Delay  SampleTime=1
  cfblk3 : DiscreteFir  SampleTime=1
  cfblk4 : slpidlib/PID Controller  Controller=PID  Form=Parallel  TimeDomain=Discrete-time  UseExternalTs=off  SampleTime=1  IntegratorMethod=Forward Euler  FilterMethod=Forward Euler  ControllerParametersSource=internal  P=1  I=1  UseKiTs=off  D=0  N=100  UseFilter=on  TunerSelectOption=Transfer Function Based (PID Tuner App)  InitialConditionSource=internal  InitialConditionForIntegrator=0  InitialConditionForFilter=0  DifferentiatorICPrevScaledInput=0  ExternalReset=none  TrackingMode=off  Kt=1  LimitOutput=off  SatLimitsSource=internal  UpperSaturationLimit=inf  LowerSaturationLimit=-inf  LinearizeAsGain=off  AntiWindupMode=none  Kb=1  LimitIntegrator=off  UpperIntegratorSaturationLimit=inf  LowerIntegratorSaturationLimit=-inf  POutMin=[]  POutMax=[]  IOutMin=[]  IOutMax=[]  DOutMin=[]  DOutMax=[]  NOutMin=[]  NOutMax=[]  SumOutMin=[]  SumOutMax=[]  SaturationOutMin=[]  SaturationOutMax=[]  PParamMin=[]  PParamMax=[]  IParamMin=[]  IParamMax=[]  DParamMin=[]  DParamMax=[]  NParamMin=[]  NParamMax=[]  KbParamMin=[]  KbParamMax=[]  KtParamMin=[]  KtParamMax=[]  KbOutMin=[]  KbOutMax=[]  KtOutMin=[]  KtOutMax=[]  IntegratorOutMin=[]  IntegratorOutMax=[]  FilterOutMin=[]  FilterOutMax=[]  SumI1OutMin=[]  SumI1OutMax=[]  SumI2OutMin=[]  SumI2OutMax=[]  SumI3OutMin=[]  SumI3OutMax=[]  SumI4OutMin=[]  SumI4OutMax=[]  SumDOutMin=[]  SumDOutMax=[]  DifferentiatorOutMin=[]  DifferentiatorOutMax=[]  FilterDiffOutCoefMin=[]  FilterDiffOutCoefMax=[]  ReciprocalOutMin=[]  ReciprocalOutMax=[]  SumDenOutMin=[]  SumDenOutMax=[]  SumNumOutMin=[]  SumNumOutMax=[]  DivideOutMin=[]  DivideOutMax=[]  UdiffTsProdOutMin=[]  UdiffTsProdOutMax=[]  NTsProdOutMin=[]  NTsProdOutMax=[]  UintegralTsProdOutMin=[]  UintegralTsProdOutMax=[]  UngainTsProdOutMin=[]  UngainTsProdOutMax=[]  ClampingZeroOutDataTypeStr=Inherit: Inherit via back propagation  ClampingZeroOutMin=[]  ClampingZeroOutMax=[]  FilterDenConstantOutDataTypeStr=Inherit: Inherit via back propagation  FilterDenConstantOutMin=[]  FilterDenConstantOutMax=[]  PCopyOutDataTypeStr=Inherit: Inherit via back propagation  PCopyOutMin=[]  PCopyOutMax=[]  NCopyOutDataTypeStr=Inherit: Inherit via back propagation  NCopyOutMin=[]  NCopyOutMax=[]  IntegratorContinuousStateAttributes=''  IntegratorStateMustResolveToSignalObject=off  IntegratorRTWStateStorageClass=Auto  FilterContinuousStateAttributes=''  FilterStateMustResolveToSignalObject=off  FilterRTWStateStorageClass=Auto  ParallelPVariant=InternalParameters  IdealPVariant=Disabled  IVariant=InternalParameters  DVariant=InternalParameters  IntegratorVariant=Discrete  SatVariant=Disabled  AWVariant=Passthrough  PCopyVariant=Disabled  TRVariant=Disabled  FdbkBlocksVariant=Forward  IdealPFdbkVariant=Disabled  SatFdbkVariant=Disabled  DerivativeFilterVariant=ForwardEulerFilter  NVariant=InternalParameters  NCopyVariant=Disabled  FilterICVariant=InternalICsFilter  IntegratorICVariant=InternalICs  ExternalResetVariant=Disabled  TRSumVariant=Passthrough  SumFdbkVariant=Disabled  SumVariant=Sum_PID  TsampFilterVariant=InternalTs  TsampNgainVariant=Passthrough  TsampIntegralVariant=Disabled_SignalSpec  ExternalSaturationOutDataTypeStr=Inherit: Same as second input
      settings: LibrarySourceBlock=simulink/Discrete/Discrete PID Controller
  cfblk5 : ComplexToRealImag
  cfblk6 : Trigonometry
  cfblk7 : Subsystem
  cfblk8 : Subsystem
  cfblk9 : Subsystem
  cfblk2 : Outport
  cfblk15 : Outport  Port=2
  cfblk16 : Outport  Port=3
  wires:
  cfblk1/1 -> cfblk5/1
  cfblk3/1 -> cfblk15/1
  cfblk4/1 -> cfblk6/1, cfblk12/3(cfblk11), cfblk12/5(cfblk13)
  cfblk6/1 -> cfblk12/1(cfblk1)
  cfblk14/1 -> cfblk16/1
  cfblk11/1(cfblk2) -> cfblk12/2(cfblk10)
  cfblk10/1(cfblk2) -> cfblk2/1
  cfblk5/1 -> cfblk11/1(cfblk1)
  cfblk12/1(cfblk2) -> cfblk3/1, cfblk10/4(cfblk11)
  cfblk5/2 -> cfblk10/2(cfblk9)
  cfblk8/2(cfblk13) -> cfblk7/1(cfblk1)
  cfblk13/1 -> cfblk11/2(cfblk13), cfblk10/5(cfblk12)
  cfblk10/2(cfblk13) -> cfblk8/2(cfblk10)
  cfblk11/2(cfblk15) -> cfblk7/2(cfblk9)
  cfblk9/2(cfblk12) -> cfblk21/1, cfblk22/1
  cfblk11/3(cfblk16) -> cfblk4/1, cfblk12/4(cfblk12)
  cfblk8/3(cfblk14) -> cfblk9/1(cfblk1)
  cfblk8/4(cfblk15) -> cfblk9/2(cfblk11)
  cfblk8/1(cfblk2) -> cfblk17/1
  cfblk17/1 -> cfblk10/1(cfblk1)
  cfblk7/1(cfblk2) -> cfblk18/1
  cfblk18/1 -> cfblk8/1(cfblk1)
  cfblk7/2(cfblk10) -> cfblk19/1
  cfblk19/1 -> cfblk10/3(cfblk10)
  cfblk9/1(cfblk2) -> cfblk20/1
  cfblk20/1 -> cfblk11/3(cfblk14)
  cfblk21/1 -> cfblk8/3(cfblk11)
  cfblk22/1 -> cfblk8/4(cfblk12)

== system model/cfblk73 ==
  cfblk1 : Inport
  cfblk11 : Inport  Port=2
  cfblk10 : Subsystem
  cfblk{13..16} (4 alike) : Delay  SampleTime=1
  cfblk3 : simulink/Discrete/Transfer Fcn Lead or Lag  PoleZ=0.95  ZeroZ=0.75  ICPrevOutput=0.0  ICPrevInput=0.0  DoSatur=off
  cfblk4 : DiscreteZeroPole  Poles=[0 0.5]  Gain=1
  cfblk5 : Sqrt
  cfblk6 : Constant  Value=[251991001.423929]  SampleTime=1
  cfblk7 : Subsystem
  cfblk8 : Subsystem
  cfblk9 : Subsystem
  cfblk2 : Outport
  cfblk12 : Outport  Port=2
  wires:
  cfblk11/1 -> cfblk10/1(cfblk1), cfblk8/4(cfblk11)
  cfblk5/1 -> cfblk13/1, cfblk14/1
  cfblk8/1(cfblk2) -> cfblk3/1
  cfblk1/1 -> cfblk7/2(cfblk13)
  cfblk4/1 -> cfblk5/1
  cfblk6/1 -> cfblk10/2(cfblk8)
  cfblk7/1(cfblk2) -> cfblk12/1
  cfblk10/1(cfblk2) -> cfblk4/1
  cfblk3/1 -> cfblk2/1, cfblk15/1
  cfblk10/2(cfblk11) -> cfblk8/1(cfblk1)
  cfblk7/2(cfblk15) -> cfblk9/1(cfblk1)
  cfblk9/1(cfblk2) -> cfblk10/3(cfblk9)
  cfblk7/3(cfblk16) -> cfblk10/4(cfblk10)
  cfblk9/2(cfblk11) -> cfblk8/2(cfblk9)
  cfblk9/3(cfblk12) -> cfblk8/3(cfblk10)
  cfblk13/1 -> cfblk7/1(cfblk1)
  cfblk14/1 -> cfblk9/2(cfblk9)
  cfblk15/1 -> cfblk9/3(cfblk10)
  cfblk8/2(cfblk12) -> cfblk16/1
  cfblk16/1 -> cfblk7/3(cfblk14)

== system model/cfblk74 ==
  cfblk1 : Inport
  cfblk5 : Inport  Port=2
  cfblk3 : DiscreteZeroPole  Poles=[0 0.5]  Gain=1
  cfblk4 : Subsystem
  cfblk2 : Outport
  cfblk6 : Outport  Port=2
  cfblk7 : Outport  Port=3
  wires:
  cfblk5/1 -> cfblk4/1(cfblk1), cfblk3/1
  cfblk1/1 -> cfblk6/1
  cfblk4/1(cfblk2) -> cfblk7/1
  cfblk3/1 -> cfblk2/1

== system model/cfblk75 ==
  cfblk1 : Inport
  cfblk5 : Inport  Port=2
  cfblk6 : Inport  Port=3
  cfblk7 : Inport  Port=4
  cfblk{10..13} (4 alike) : Delay  SampleTime=1
  cfblk3 : Subsystem
  cfblk4 : If  IfExpression=u1 >= 0  SampleTime=1
  cfblk8 : Subsystem  TreatAsAtomicUnit=on
  cfblk9 : Subsystem  TreatAsAtomicUnit=on
  cfblk2 : Outport
  wires:
  cfblk5/1 -> cfblk9/1(cfblk1)
  cfblk7/1 -> cfblk4/1
  cfblk1/1 -> cfblk3/1(cfblk1)
  cfblk6/1 -> cfblk8/1(cfblk1)
  cfblk3/1(cfblk2) -> cfblk9/2(cfblk13)
  cfblk9/1(cfblk2) -> cfblk8/2(cfblk10)
  cfblk9/3(cfblk15) -> cfblk8/3(cfblk11)
  cfblk9/4(cfblk16) -> cfblk12/1, cfblk13/1
  cfblk8/1(cfblk2) -> cfblk2/1
  cfblk3/2(cfblk17) -> cfblk8/4(cfblk12)
  cfblk4/1 -> cfblk8/Action
  cfblk4/2 -> cfblk9/Action
  cfblk8/2(cfblk13) -> cfblk10/1
  cfblk10/1 -> cfblk3/4(cfblk15)
  cfblk9/2(cfblk14) -> cfblk11/1
  cfblk11/1 -> cfblk3/2(cfblk13)
  cfblk12/1 -> cfblk3/3(cfblk14)
  cfblk13/1 -> cfblk3/5(cfblk16)

== system model/cfblk76 ==
  cfblk1 : Inport
  cfblk13 : Inport  Port=2
  cfblk14 : Inport  Port=3
  cfblk10 : Subsystem
  cfblk11 : Subsystem
  cfblk12 : Subsystem
  cfblk15 : Delay  SampleTime=1
  cfblk16 : Delay  SampleTime=1
  cfblk3 : simulink/Discrete/Tapped Delay  vinit=0.0  samptime=-1  NumDelays=1  DelayOrder=Oldest  includeCurrent=off
  cfblk4 : simulink/Discrete/Difference  ICPrevInput=0.0  OutMin=[]  OutMax=[]  OutDataTypeStr=Inherit: Inherit via back propagation  OutDataType=fixdt(1, 16)  OutScaling=2^-10  DoSatur=off
  cfblk5 : DiscreteZeroPole  Poles=[0 0.5]  Gain=1
  cfblk6 : simulink/Math Operations/Slider Gain  gain=1  low=0  high=2
  cfblk7 : UnaryMinus
  cfblk8 : PermuteDimensions
  cfblk9 : Subsystem
  cfblk2 : Outport
  wires:
  cfblk7/1 -> cfblk12/1(cfblk1)
  cfblk8/1 -> cfblk10/1(cfblk1)
  cfblk4/1 -> cfblk2/1
  cfblk1/1 -> cfblk9/1(cfblk1)
  cfblk3/1 -> cfblk12/3(cfblk8)
  cfblk13/1 -> cfblk10/2(cfblk7)
  cfblk11/1(cfblk2) -> cfblk5/1
  cfblk14/1 -> cfblk7/1
  cfblk12/1(cfblk2) -> cfblk8/1
  cfblk10/2(cfblk8) -> cfblk11/1(cfblk1)
  cfblk6/1 -> cfblk4/1
  cfblk11/3(cfblk7) -> cfblk6/1
  cfblk10/1(cfblk2) -> cfblk15/1
  cfblk15/1 -> cfblk12/2(cfblk7)
  cfblk11/2(cfblk6) -> cfblk16/1
  cfblk16/1 -> cfblk3/1

== system model/cfblk77 ==
  cfblk1 : Inport
  cfblk10 : Subsystem
  cfblk11 : Subsystem
  cfblk{13..17} (5 alike) : Delay  SampleTime=1
  cfblk3 : Delay  ShowEnablePort=on  SampleTime=1
      settings: InputPortMap=u0,e6
  cfblk4 : UnaryMinus
  cfblk5 : MinMax  Function=max
  cfblk6 : Sqrt
  cfblk7 : simulink/Math Operations/MinMax Running Resettable  Function=min  vinit=0.0
  cfblk8 : Subsystem
  cfblk9 : Subsystem
  cfblk2 : Outport
  cfblk12 : Outport  Port=2
  wires:
  cfblk10/1(cfblk2) -> cfblk2/1
  cfblk9/1(cfblk2) -> cfblk3/1
  cfblk11/1(cfblk2) -> cfblk6/1
  cfblk6/1 -> cfblk8/1(cfblk1), cfblk16/1
  cfblk1/1 -> cfblk9/2(cfblk11)
  cfblk4/1 -> cfblk5/1
  cfblk10/2(cfblk11) -> cfblk11/1(cfblk1)
  cfblk9/2(cfblk13) -> cfblk3/2
  cfblk11/2(cfblk7) -> cfblk8/2(cfblk12), cfblk7/1
  cfblk10/3(cfblk12) -> cfblk4/1, cfblk12/1
  cfblk3/1 -> cfblk10/4(cfblk10), cfblk13/1
  cfblk8/1(cfblk2) -> cfblk7/2, cfblk14/1
  cfblk13/1 -> cfblk9/3(cfblk12)
  cfblk14/1 -> cfblk10/2(cfblk8)
  cfblk7/1 -> cfblk15/1
  cfblk15/1 -> cfblk10/1(cfblk1)
  cfblk16/1 -> cfblk10/3(cfblk9)
  cfblk5/1 -> cfblk17/1
  cfblk17/1 -> cfblk9/1(cfblk1)

== system model/cfblk78 ==
  cfblk1 : Inport
  cfblk3 : Delay  SampleTime=1
  cfblk4 : Reshape
  cfblk5 : Sum  Inputs=+
  cfblk6 : Subsystem
  cfblk7 : Subsystem
  cfblk8 : Delay  SampleTime=1
  cfblk2 : Outport
  wires:
  cfblk1/1 -> cfblk4/1
  cfblk7/1(cfblk2) -> cfblk6/1(cfblk1)
  cfblk4/1 -> cfblk5/1, cfblk6/3(cfblk9)
  cfblk6/1(cfblk2) -> cfblk2/1
  cfblk5/1 -> cfblk7/2(cfblk8)
  cfblk7/2(cfblk9) -> cfblk3/1
  cfblk3/1 -> cfblk6/2(cfblk8)
  cfblk6/2(cfblk10) -> cfblk8/1
  cfblk8/1 -> cfblk7/1(cfblk1)

== system model/cfblk79 ==
  cfblk1 : Inport
  cfblk14 : Inport  Port=2
  cfblk10 : Subsystem
  cfblk11 : Subsystem
  cfblk12 : Subsystem
  cfblk13 : Subsystem
  cfblk15 : Delay  SampleTime=1
  cfblk16 : Delay  SampleTime=1
  cfblk3 : simulink/Discrete/Difference  ICPrevInput=0.0  OutMin=[]  OutMax=[]  OutDataTypeStr=Inherit: Inherit via back propagation  OutDataType=fixdt(1, 16)  OutScaling=2^-10  DoSatur=off
  cfblk4 : Delay  DelayLengthSource=Input port  SampleTime=1
      settings: InputPortMap=u0,p1
  cfblk5 : Delay  ShowEnablePort=on  SampleTime=1
      settings: InputPortMap=u0,e6
  cfblk6 : Delay  ShowEnablePort=on  SampleTime=1
      settings: InputPortMap=u0,e6
  cfblk7 : Gain  Gain=[-633947602.308004]
  cfblk8 : Constant  Value=[6845603.135488]  SampleTime=1
  cfblk9 : Subsystem
  cfblk2 : Outport
  wires:
  cfblk13/1(cfblk2) -> cfblk6/1
  cfblk8/1 -> cfblk12/1(cfblk1)
  cfblk5/1 -> cfblk7/1
  cfblk4/1 -> cfblk11/1(cfblk1), cfblk9/2(cfblk4), cfblk9/3(cfblk5)
  cfblk10/1(cfblk2) -> cfblk5/1
  cfblk6/1 -> cfblk9/5(cfblk7), cfblk16/1
  cfblk14/1 -> cfblk3/1, cfblk9/1(cfblk1)
  cfblk9/1(cfblk2) -> cfblk10/1(cfblk1)
  cfblk12/1(cfblk2) -> cfblk2/1
  cfblk3/1 -> cfblk6/2
  cfblk11/1(cfblk2) -> cfblk10/2(cfblk7), cfblk13/1(cfblk1)
  cfblk12/2(cfblk8) -> cfblk4/1, cfblk9/4(cfblk6)
  cfblk1/1 -> cfblk4/2
  cfblk7/1 -> cfblk15/1
  cfblk15/1 -> cfblk5/2
  cfblk16/1 -> cfblk11/2(cfblk7)

== system model/cfblk80 ==
  cfblk1 : Inport
  cfblk7 : Inport  Port=2
  cfblk3 : DiscreteFilter  SampleTime=1
  cfblk4 : ComplexToRealImag
  cfblk5 : Constant  Value=[-268454467.432629]  SampleTime=1
  cfblk6 : Subsystem
  cfblk8 : Delay  SampleTime=1
  cfblk2 : Outport
  wires:
  cfblk7/1 -> cfblk2/1
  cfblk5/1 -> cfblk4/1
  cfblk4/1 -> cfblk6/2(cfblk14)
  cfblk1/1 -> cfblk6/3(cfblk15)
  cfblk4/2 -> cfblk6/4(cfblk16)
  cfblk6/1(cfblk2) -> cfblk3/1
  cfblk3/1 -> cfblk8/1
  cfblk8/1 -> cfblk6/1(cfblk1)

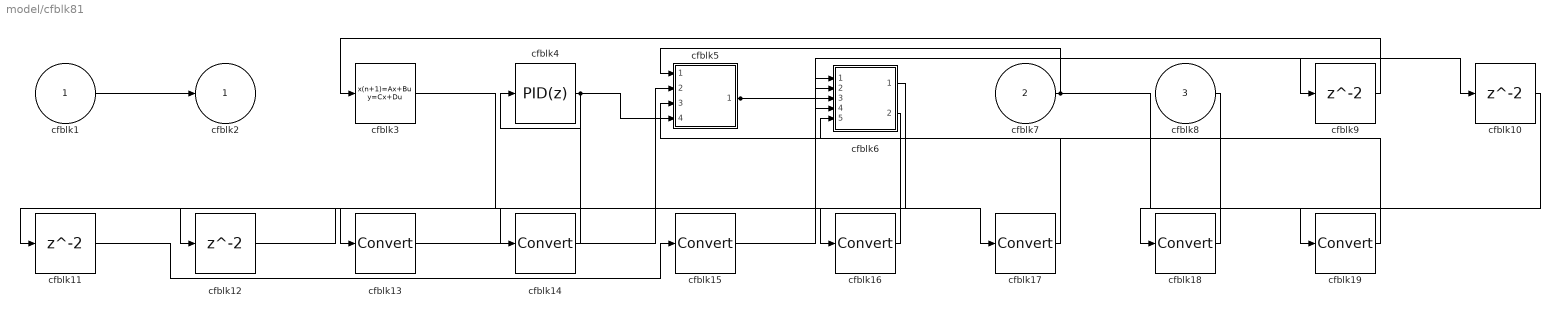
== system model/cfblk81 ==
  cfblk1 : Inport
  cfblk7 : Inport  Port=2
  cfblk8 : Inport  Port=3
  cfblk{9..12} (4 alike) : Delay  SampleTime=1
  cfblk{13..19} (7 alike) : DataTypeConversion  SaturateOnIntegerOverflow=off  RndMeth=Floor
  cfblk3 : DiscreteStateSpace
  cfblk4 : slpidlib/PID Controller  Controller=PID  Form=Parallel  TimeDomain=Discrete-time  UseExternalTs=off  SampleTime=1  IntegratorMethod=Forward Euler  FilterMethod=Forward Euler  ControllerParametersSource=internal  P=1  I=1  UseKiTs=off  D=0  N=100  UseFilter=on  TunerSelectOption=Transfer Function Based (PID Tuner App)  InitialConditionSource=internal  InitialConditionForIntegrator=0  InitialConditionForFilter=0  DifferentiatorICPrevScaledInput=0  ExternalReset=none  TrackingMode=off  Kt=1  LimitOutput=off  SatLimitsSource=internal  UpperSaturationLimit=inf  LowerSaturationLimit=-inf  LinearizeAsGain=off  AntiWindupMode=none  Kb=1  LimitIntegrator=off  UpperIntegratorSaturationLimit=inf  LowerIntegratorSaturationLimit=-inf  POutMin=[]  POutMax=[]  IOutMin=[]  IOutMax=[]  DOutMin=[]  DOutMax=[]  NOutMin=[]  NOutMax=[]  SumOutMin=[]  SumOutMax=[]  SaturationOutMin=[]  SaturationOutMax=[]  PParamMin=[]  PParamMax=[]  IParamMin=[]  IParamMax=[]  DParamMin=[]  DParamMax=[]  NParamMin=[]  NParamMax=[]  KbParamMin=[]  KbParamMax=[]  KtParamMin=[]  KtParamMax=[]  KbOutMin=[]  KbOutMax=[]  KtOutMin=[]  KtOutMax=[]  IntegratorOutMin=[]  IntegratorOutMax=[]  FilterOutMin=[]  FilterOutMax=[]  SumI1OutMin=[]  SumI1OutMax=[]  SumI2OutMin=[]  SumI2OutMax=[]  SumI3OutMin=[]  SumI3OutMax=[]  SumI4OutMin=[]  SumI4OutMax=[]  SumDOutMin=[]  SumDOutMax=[]  DifferentiatorOutMin=[]  DifferentiatorOutMax=[]  FilterDiffOutCoefMin=[]  FilterDiffOutCoefMax=[]  ReciprocalOutMin=[]  ReciprocalOutMax=[]  SumDenOutMin=[]  SumDenOutMax=[]  SumNumOutMin=[]  SumNumOutMax=[]  DivideOutMin=[]  DivideOutMax=[]  UdiffTsProdOutMin=[]  UdiffTsProdOutMax=[]  NTsProdOutMin=[]  NTsProdOutMax=[]  UintegralTsProdOutMin=[]  UintegralTsProdOutMax=[]  UngainTsProdOutMin=[]  UngainTsProdOutMax=[]  ClampingZeroOutDataTypeStr=Inherit: Inherit via back propagation  ClampingZeroOutMin=[]  ClampingZeroOutMax=[]  FilterDenConstantOutDataTypeStr=Inherit: Inherit via back propagation  FilterDenConstantOutMin=[]  FilterDenConstantOutMax=[]  PCopyOutDataTypeStr=Inherit: Inherit via back propagation  PCopyOutMin=[]  PCopyOutMax=[]  NCopyOutDataTypeStr=Inherit: Inherit via back propagation  NCopyOutMin=[]  NCopyOutMax=[]  IntegratorContinuousStateAttributes=''  IntegratorStateMustResolveToSignalObject=off  IntegratorRTWStateStorageClass=Auto  FilterContinuousStateAttributes=''  FilterStateMustResolveToSignalObject=off  FilterRTWStateStorageClass=Auto  ParallelPVariant=InternalParameters  IdealPVariant=Disabled  IVariant=InternalParameters  DVariant=InternalParameters  IntegratorVariant=Discrete  SatVariant=Disabled  AWVariant=Passthrough  PCopyVariant=Disabled  TRVariant=Disabled  FdbkBlocksVariant=Forward  IdealPFdbkVariant=Disabled  SatFdbkVariant=Disabled  DerivativeFilterVariant=ForwardEulerFilter  NVariant=InternalParameters  NCopyVariant=Disabled  FilterICVariant=InternalICsFilter  IntegratorICVariant=InternalICs  ExternalResetVariant=Disabled  TRSumVariant=Passthrough  SumFdbkVariant=Disabled  SumVariant=Sum_PID  TsampFilterVariant=InternalTs  TsampNgainVariant=Passthrough  TsampIntegralVariant=Disabled_SignalSpec  ExternalSaturationOutDataTypeStr=Inherit: Same as second input
      settings: LibrarySourceBlock=simulink/Discrete/Discrete PID Controller
  cfblk5 : Subsystem
  cfblk6 : Subsystem
  cfblk2 : Outport
  wires:
  cfblk4/1 -> cfblk5/4(cfblk9), cfblk11/1, cfblk12/1
  cfblk1/1 -> cfblk2/1
  cfblk7/1 -> cfblk5/1(cfblk1), cfblk19/1
  cfblk8/1 -> cfblk5/3(cfblk8)
  cfblk5/1(cfblk2) -> cfblk9/1, cfblk10/1
  cfblk9/1 -> cfblk3/1
  cfblk6/1(cfblk2) -> cfblk13/1
  cfblk13/1 -> cfblk5/2(cfblk7)
  cfblk6/2(cfblk12) -> cfblk14/1
  cfblk14/1 -> cfblk4/1
  cfblk11/1 -> cfblk15/1
  cfblk15/1 -> cfblk6/1(cfblk1)
  cfblk3/1 -> cfblk16/1
  cfblk16/1 -> cfblk6/2(cfblk8)
  cfblk12/1 -> cfblk17/1
  cfblk17/1 -> cfblk6/3(cfblk9)
  cfblk10/1 -> cfblk18/1
  cfblk18/1 -> cfblk6/4(cfblk10)
  cfblk19/1 -> cfblk6/5(cfblk11)

== system model/cfblk82 ==
  cfblk1 : Inport
  cfblk9 : Inport  Port=2
  cfblk10 : Inport  Port=3
  cfblk11 : Delay  SampleTime=1
  cfblk12 : Delay  SampleTime=1
  cfblk3 : Subsystem
  cfblk4 : Subsystem
  cfblk5 : Subsystem
  cfblk6 : Subsystem
  cfblk7 : Subsystem
  cfblk8 : Subsystem
  cfblk2 : Outport
  wires:
  cfblk6/1(cfblk2) -> cfblk2/1
  cfblk9/1 -> cfblk4/1(cfblk1)
  cfblk1/1 -> cfblk5/2(cfblk9)
  cfblk4/1(cfblk2) -> cfblk3/1(cfblk1)
  cfblk5/1(cfblk2) -> cfblk8/1(cfblk1)
  cfblk5/2(cfblk11) -> cfblk8/2(cfblk13)
  cfblk4/2(cfblk13) -> cfblk7/1(cfblk1)
  cfblk7/1(cfblk2) -> cfblk3/2(cfblk16)
  cfblk8/2(cfblk14) -> cfblk6/1(cfblk1)
  cfblk10/1 -> cfblk5/3(cfblk10)
  cfblk6/2(cfblk9) -> cfblk7/2(cfblk8)
  cfblk8/1(cfblk2) -> cfblk11/1
  cfblk11/1 -> cfblk5/1(cfblk1)
  cfblk3/1(cfblk2) -> cfblk12/1
  cfblk12/1 -> cfblk7/3(cfblk9)

== system model/cfblk83 ==
  cfblk1 : Inport
  cfblk10 : Inport  Port=2
  cfblk12 : Delay  SampleTime=1
  cfblk13 : Delay  SampleTime=1
  cfblk3 : DiscreteIntegrator  ICPrevOutput=DiscIntNeverNeededParam  ICPrevScaledInput=DiscIntNeverNeededParam
  cfblk4 : DiscreteStateSpace
  cfblk5 : Sqrt
  cfblk6 : PermuteDimensions
  cfblk7 : Reshape
  cfblk8 : Squeeze
  cfblk9 : Subsystem
  cfblk2 : Outport
  cfblk11 : Outport  Port=2
  wires:
  cfblk4/1 -> cfblk8/1
  cfblk3/1 -> cfblk5/1
  cfblk1/1 -> cfblk11/1
  cfblk9/1(cfblk2) -> cfblk4/1
  cfblk10/1 -> cfblk2/1
  cfblk9/2(cfblk11) -> cfblk6/1
  cfblk5/1 -> cfblk9/2(cfblk10)
  cfblk6/1 -> cfblk7/1
  cfblk8/1 -> cfblk12/1
  cfblk12/1 -> cfblk3/1
  cfblk7/1 -> cfblk13/1
  cfblk13/1 -> cfblk9/1(cfblk1)

== system model/cfblk84 ==
  cfblk1 : Inport
  cfblk10 : Delay  SampleTime=1
  cfblk11 : Delay  SampleTime=1
  cfblk3 : simulink/Discrete/Transfer Fcn Real Zero  ZeroZ=0.75  ICPrevInput=0.0  DoSatur=off
  cfblk4 : UnaryMinus
  cfblk5 : Constant  Value=[-837861540.979902]  SampleTime=1
  cfblk6 : Subsystem
  cfblk7 : Subsystem
  cfblk8 : Subsystem
  cfblk9 : Delay  SampleTime=1
  cfblk2 : Outport
  wires:
  cfblk5/1 -> cfblk2/1
  cfblk6/1(cfblk2) -> cfblk8/1(cfblk1)
  cfblk3/1 -> cfblk4/1
  cfblk4/1 -> cfblk6/2(cfblk11)
  cfblk8/3(cfblk14) -> cfblk7/1(cfblk1)
  cfblk6/2(cfblk13) -> cfblk7/2(cfblk7)
  cfblk8/4(cfblk15) -> cfblk7/3(cfblk8)
  cfblk6/3(cfblk14) -> cfblk7/4(cfblk9)
  cfblk8/1(cfblk2) -> cfblk9/1
  cfblk9/1 -> cfblk3/1
  cfblk8/2(cfblk13) -> cfblk10/1
  cfblk10/1 -> cfblk6/3(cfblk12)
  cfblk7/1(cfblk2) -> cfblk11/1
  cfblk11/1 -> cfblk6/1(cfblk1)

== system model/cfblk85 ==
  cfblk1 : Inport
  cfblk10 : Subsystem
  cfblk11 : Subsystem
  cfblk13 : Delay  SampleTime=1
  cfblk14 : Delay  SampleTime=1
  cfblk15 : Delay  SampleTime=1
  cfblk3 : simulink/Discrete/Transfer Fcn Lead or Lag  PoleZ=0.95  ZeroZ=0.75  ICPrevOutput=0.0  ICPrevInput=0.0  DoSatur=off
  cfblk4 : DiscreteFir  SampleTime=1
  cfblk5 : Trigonometry
  cfblk6 : simulink/Math Operations/Slider Gain  gain=1  low=0  high=2
  cfblk7 : simulink/Math Operations/MinMax Running Resettable  Function=min  vinit=0.0
  cfblk8 : MinMax  Inputs=2
  cfblk9 : Constant  Value=[36903658.818854]  SampleTime=1
  cfblk2 : Outport
  cfblk12 : Outport  Port=2
  wires:
  cfblk7/1 -> cfblk6/1, cfblk12/1
  cfblk9/1 -> cfblk11/1(cfblk1)
  cfblk10/1(cfblk2) -> cfblk11/2(cfblk12)
  cfblk8/1 -> cfblk2/1
  cfblk11/1(cfblk2) -> cfblk8/1
  cfblk4/1 -> cfblk8/2, cfblk13/1, cfblk14/1
  cfblk5/1 -> cfblk4/1
  cfblk10/2(cfblk7) -> cfblk5/1
  cfblk3/1 -> cfblk10/2(cfblk5), cfblk7/2
  cfblk1/1 -> cfblk3/1
  cfblk13/1 -> cfblk10/1(cfblk1)
  cfblk14/1 -> cfblk10/3(cfblk6)
  cfblk6/1 -> cfblk15/1
  cfblk15/1 -> cfblk7/1

== system model/cfblk91 ==
  cfblk1 : Inport
  cfblk7 : Inport  Port=2
  Action Port : ActionPort  ActionPortLabel=if(u1 >= 0)
  cfblk10 : Delay
  cfblk11 : Delay
  cfblk3 : Rounding
  cfblk4 : Subsystem
  cfblk5 : Subsystem
  cfblk6 : Subsystem
  cfblk2 : Outport
  cfblk8 : Outport  Port=2
  cfblk9 : Outport  Port=3
  wires:
  cfblk7/1 -> cfblk6/1(cfblk1)
  cfblk4/1(cfblk2) -> cfblk9/1
  cfblk3/1 -> cfblk10/1, cfblk11/1
  cfblk5/1(cfblk2) -> cfblk3/1
  cfblk6/1(cfblk2) -> cfblk2/1, cfblk5/1(cfblk1), cfblk8/1, cfblk5/2(cfblk15), cfblk5/3(cfblk16), cfblk4/3(cfblk12), cfblk4/5(cfblk14)
  cfblk1/1 -> cfblk4/1(cfblk1), cfblk6/4(cfblk16), cfblk6/5(cfblk17), cfblk4/2(cfblk11), cfblk4/4(cfblk13)
  cfblk10/1 -> cfblk6/2(cfblk14)
  cfblk11/1 -> cfblk6/3(cfblk15)
